simulink model "mode_selector"  (R2021a)
settings: Solver=FixedStepDiscrete  StartTime=0.0  StopTime=10.0  FixedStep=0.1  RelTol=1e-3  EnableMultiTasking=on
settings Model: Creator=afonso.miguel  LastModifiedBy=afonso.miguel
settings SolverCC: AlgebraicLoopSolver=TrustRegion  AutoInsertRateTranBlk=on
settings DataIOCC: LimitDataPoints=on
settings OptimizationCC: LifeSpan=inf
settings DebuggingCC: AllowSymbolicDim=off  SFUnexpectedBacktrackingDiag=warning  SFNoUnconditionalDefaultTransitionDiag=warning  SFExecutionAtInitializationDiag=none  ArithmeticOperatorsInVariantConditions=warning
settings SFSimCC: SimUseLocalCustomCode=off  CustomCodeUndefinedFunction=UseInterfaceOnly
settings RTWCC: RTWUseLocalCustomCode=off
settings CodeAppCC: StateflowObjectComments=on
settings GRTTargetCC: TargetLangStandard=C89/C90 (ANSI)
settings ConfigComp: CovMetricSettings=dw  CovSaveCumulativeToWorkspaceVar=on  CovSaveSingleToWorkspaceVar=on  CovExternalEMLEnable=off  CovSFcnEnable=off

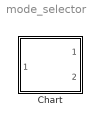
== system mode_selector ==
  Chart : Stateflow chart  TreatAsAtomicUnit=on

== stateflow chart mode_selector/Chart ==
  settings: executeAtInitialization=1
  state init
  state WaitingChange
  state Step1
  state Step2
  (default) -> init
  init -> WaitingChange : {mode=0; changing=1;}
  Step2 -> WaitingChange [order 2] : {mode=mode_buffer2}
  WaitingChange -> WaitingChange [order 1] : [mode_in==mode]
      | {changing=0}
  Step1 -> WaitingChange [order 1] : [mode_in~=mode_buffer1]
  Step2 -> WaitingChange [order 1] : [mode_in~=mode_buffer2]
  WaitingChange -> Step1 [order 2] : {mode_buffer1=mode;
      | changing=1;}
  Step1 -> Step2 [order 2] : {mode_buffer2=mode;}
  data: mode output fixdt(0,1,0); mode_in input fixdt(0,2,0); mode_buffer1 local fixdt(0,2,0); mode_buffer2 local fixdt(0,2,0); changing output
